simulink model "zad8disc_lin"  (R2014b)
settings: Solver=ode45  StartTime=0.0  StopTime=50  RelTol=1e-3
values from neighbouring files (symbols this model uses):
  a1 = -0.28    [set_params.m]
  a2 = -0.9    [set_params.m]
  a3 = 0.35    [set_params.m]
  a4 = 0.3    [set_params.m]
  K = 4.5    [set_params.m]
  selector = 0    [zad9.m]
  T1 = 5    [set_params.m]
  T2 = 8    [set_params.m]
  Tp = 1    [zad10.m]    (also in zad11.m; zad3.m = Tp_vect(i); zad9.m)
  u_lin = linspace(-1,1,101)    [zad11.m]    (also in zad12.m = 1; zad6.m = K*a1*u + K*(a2*(u_p^2) + a3*(u_p^3) + a4*(u_p^4)) + K*(u - u; zad9.m = pkt_lin(i))
libraries: simulink x3
settings Model: Creator=kuba  LastModifiedBy=kuba

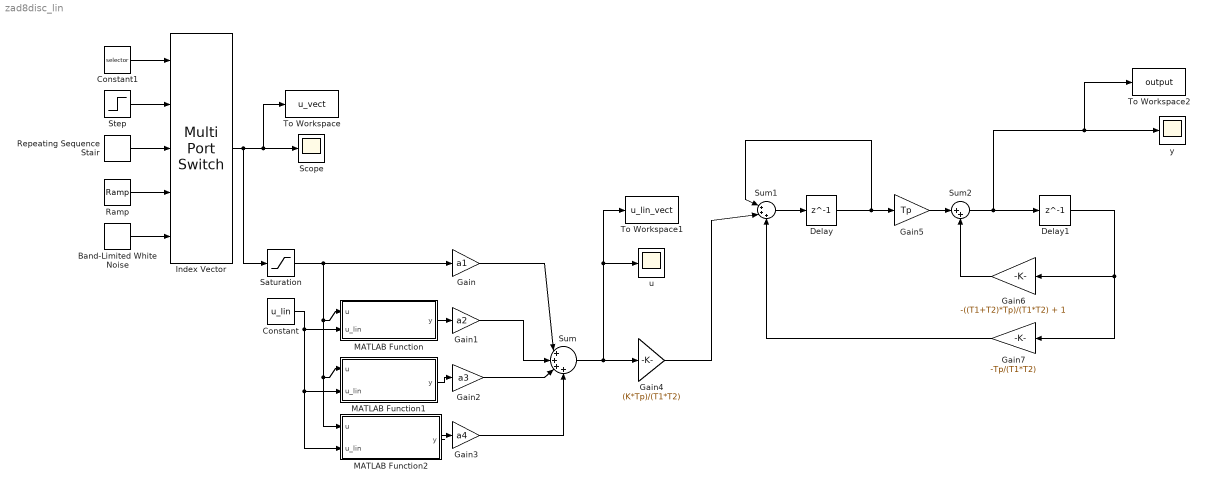
== system zad8disc_lin ==
  Band-Limited White Noise : simulink/Sources/Band-Limited White Noise  Cov=[0.1]  Ts=0.1  seed=[23341]
  Constant : Constant  Value=u_lin  SampleTime=Tp
  Constant1 : Constant  Value=selector
  Delay : Delay  DelayLength=1  SampleTime=Tp
  Delay1 : Delay  DelayLength=1  SampleTime=Tp
  Gain : Gain  Gain=a1  SampleTime=Tp
  Gain1 : Gain  Gain=a2  SampleTime=Tp
  Gain2 : Gain  Gain=a3  SampleTime=Tp
  Gain3 : Gain  Gain=a4  SampleTime=Tp
  Gain4 : Gain  Gain=(K*Tp)/(T1*T2)
  Gain5 : Gain  Gain=Tp
  Gain6 : Gain  Gain=-((T1+T2)*Tp)/(T1*T2) + 1
  Gain7 : Gain  Gain=-Tp/(T1*T2)
  Index Vector : MultiPortSwitch  DataPortOrder=Zero-based contiguous  Inputs=4  zeroidx=on
  MATLAB Function : MATLAB Function  TreatAsAtomicUnit=on
  MATLAB Function1 : MATLAB Function  TreatAsAtomicUnit=on
  MATLAB Function2 : MATLAB Function  TreatAsAtomicUnit=on
  Ramp : simulink/Sources/Ramp  slope=0.05  start=0  X0=0
  Repeating Sequence Stair : simulink/Sources/Repeating Sequence Stair  OutValues=[0.4 0.8 1 0.4 -0.2 -0.6 -1 -0.6].'  tsamp=5  OutMin=[]  OutMax=[]  OutDataTypeStr=double  OutputDataTypeScalingMode=double  OutDataType=fixdt(0,8)  ConRadixGroup=Best Precision: Vector-wise  OutScaling=2^-12
  Saturation : Saturate  UpperLimit=1  LowerLimit=-1
  Scope : Scope
      settings: TimeRange=50  YMin=-1  YMax=1  SaveName=ScopeData2
  Step : Step  SampleTime=0
  Sum : Sum  Inputs=|++++
  Sum1 : Sum  Inputs=|+++
  Sum2 : Sum  Inputs=|++
  To Workspace : ToWorkspace  VariableName=u_vect  SaveFormat=Timeseries  SampleTime=-1
  To Workspace1 : ToWorkspace  VariableName=u_lin_vect  SaveFormat=Timeseries  SampleTime=-1
  To Workspace2 : ToWorkspace  VariableName=output  SaveFormat=Timeseries  SampleTime=-1
  u : Scope
  y : Scope
      settings: TimeRange=100  YMin=-1  YMax=1
  wires:
  Saturation/1 -> MATLAB Function2/1(u), MATLAB Function1/1(u), MATLAB Function/1(u), Gain/1
  MATLAB Function/1(y) -> Gain1/1
  MATLAB Function1/1(y) -> Gain2/1
  MATLAB Function2/1(y) -> Gain3/1
  Gain/1 -> Sum/1
  Gain1/1 -> Sum/2
  Gain2/1 -> Sum/3
  Gain3/1 -> Sum/4
  Sum/1 -> To Workspace1/1, u/1, Gain4/1
  Gain4/1 -> Sum1/2
  Sum1/1 -> Delay/1
  Delay/1 -> Gain5/1, Sum1/1
  Gain5/1 -> Sum2/1
  Sum2/1 -> To Workspace2/1, y/1, Delay1/1
  Gain6/1 -> Sum2/2
  Gain7/1 -> Sum1/3
  Delay1/1 -> Gain7/1, Gain6/1
  Constant/1 -> MATLAB Function2/2(u_lin), MATLAB Function1/2(u_lin), MATLAB Function/2(u_lin)
  Band-Limited White Noise/1 -> Index Vector/5
  Ramp/1 -> Index Vector/4
  Index Vector/1 -> Saturation/1, To Workspace/1, Scope/1
  Step/1 -> Index Vector/2
  Repeating Sequence Stair/1 -> Index Vector/3
  Constant1/1 -> Index Vector/1

== matlab function zad8disc_lin/MATLAB Function1 ==
  data: u input; y output; u_lin input
function y = cube_lin(u, u_lin)
y = u_lin^3 + 3*(u_lin^2)*(u-u_lin);

== matlab function zad8disc_lin/MATLAB Function ==
  data: u input; y output; u_lin input
function y = square_lin(u, u_lin)
y = u_lin.^2 + 2*u_lin*(u - u_lin);

== matlab function zad8disc_lin/MATLAB Function2 ==
  data: u input; y output; u_lin input
function y = quad_lin(u, u_lin)
y = u_lin^4 + 4*(u_lin^3)*(u - u_lin);
